simulink model "Series_Connection_Thyristor_Simulink"  (R2021b)
settings: Solver=VariableStepAuto  StartTime=0.0  StopTime=0.005  RelTol=1e-3
undefined symbols (not defined in the file): Ts
libraries: spsThyristorLib x2, spsDCVoltageSourceLib x1, spsSeriesRLCBranchLib x1, spsVoltageMeasurementLib x1, spspowerguiLib x1
settings Model: Creator=Vansh  LastModifiedBy=Vansh

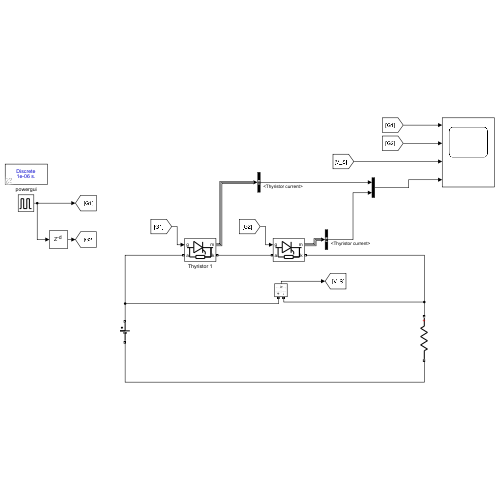
[thumbnail: Simulink's stored preview of the top-level diagram]
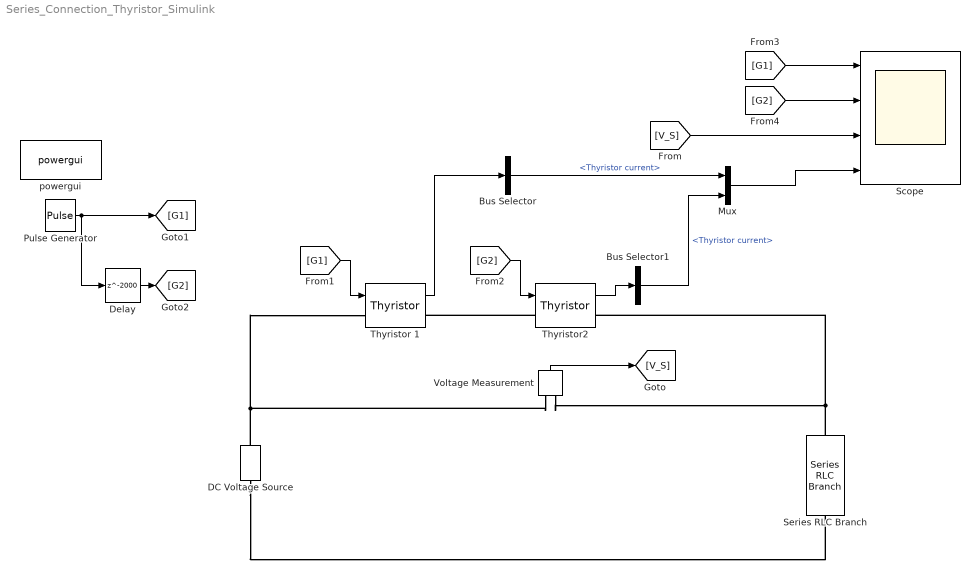
== system Series_Connection_Thyristor_Simulink ==
  Bus Selector : BusSelector  OutputSignals=Thyristor current
  Bus Selector1 : BusSelector  OutputSignals=Thyristor current
  DC Voltage Source : spsDCVoltageSourceLib/DC Voltage Source  Amplitude=100  Measurements=None
  Delay : Delay  DelayLength=2000  SampleTime=Ts
  Mux : Mux  Inputs=2
  Pulse Generator : DiscretePulseGenerator  PulseType=Time based  Period=0.005  PulseWidth=5  PhaseDelay=0.001
  Scope : Scope  NumInputPorts=4
  Series RLC Branch : spsSeriesRLCBranchLib/Series RLC Branch  LConnTagsString=__new0  RConnTagsString=__new0  BranchType=R  Resistance=10  Inductance=1e-3  SetiL0=off  InitialCurrent=0  Capacitance=1e-6  Setx0=off  InitialVoltage=0  Measurements=None
  Thyristor 1 : spsThyristorLib/Thyristor  Ron=0.001  Lon=0  Vf=0.8  IC=0  Rs=500  Cs=250e-9  Measurements=on
  Thyristor2 : spsThyristorLib/Thyristor  Ron=0.001  Lon=0  Vf=0.8  IC=0  Rs=500  Cs=250e-9  Measurements=on
  Voltage Measurement : spsVoltageMeasurementLib/Voltage Measurement  PhasorSimulation=off  OutputType=Complex  PSBequivalent=0
  powergui : spspowerguiLib/powergui  Priority=1  SimulationMode=Discrete  SampleTime=Ts  frequency=60  Iterations=50  frequencyindice=0  Pbase=100e6  ErrMax=1e-4  UnitsV=kV  UnitsW=MW  buscounter=0  FunctionMessages=off  echomessages=off  EnableUseOfTLC=off  CurrentSourceSwitches=off  DisableSnubberDevices=off  DisableRonSwitches=off  DisableVfSwitches=off  DisplayEquations=off  AutomaticDiscreteSolvers=off  SolverType=Tustin/Backward Euler (TBE)  Interpol=off  ExternalGateDelay=off  methode=off  Ts=100  x0status=blocks  SPID=on  SwTol=0  HookPort=off  NonlinearTolerance=1e-4  nMaxIteration=100  ContinueOnMaxIteration=off  RestoreLinks=warning  ResistiveCurrentMeasurement=off  Frange=[0:2:500]  Ylog=off  Xlog=on  ShowGrid=off  save=off  variable=ZData  structure=0  ZoomFFT=off  StartTime=0.0  cycles=1  DisplayStyle=1  fundamental=60  FreqAxis=off  MaxFrequency=1000  frequencyindicesteady=1  RmsSteady=1  display=off
  wires:
  [G2] -> Thyristor2/1
  Thyristor 1/1 -> Bus Selector/1
  Thyristor2/1 -> Bus Selector1/1
  Bus Selector1/1 -> Mux/2  "<Thyristor current>"
  Mux/1 -> Scope/4
  [V_S] -> Scope/3
  Pulse Generator/1 -> [G1], Delay/1
  [G1] -> Thyristor 1/1
  Delay/1 -> [G2]
  [G1] -> Scope/1
  [G2] -> Scope/2
  Bus Selector/1 -> Mux/1  "<Thyristor current>"
  Voltage Measurement/1 -> [V_S]
  connections:
  DC Voltage Source/RConn1 -- Voltage Measurement/LConn1 -- Thyristor 1/LConn1
  Series RLC Branch/LConn1 -- Thyristor2/RConn1 -- Voltage Measurement/LConn2
  DC Voltage Source/LConn1 -- Series RLC Branch/RConn1
  Thyristor2/LConn1 -- Thyristor 1/RConn1
